simulink model "elec3200lab2"  (R2016a)
settings: Solver=VariableStepAuto  StartTime=0.0  StopTime=2  RelTol=1e-3
libraries: simulink x1
settings Model: Creator=古乔  LastModifiedBy=古乔

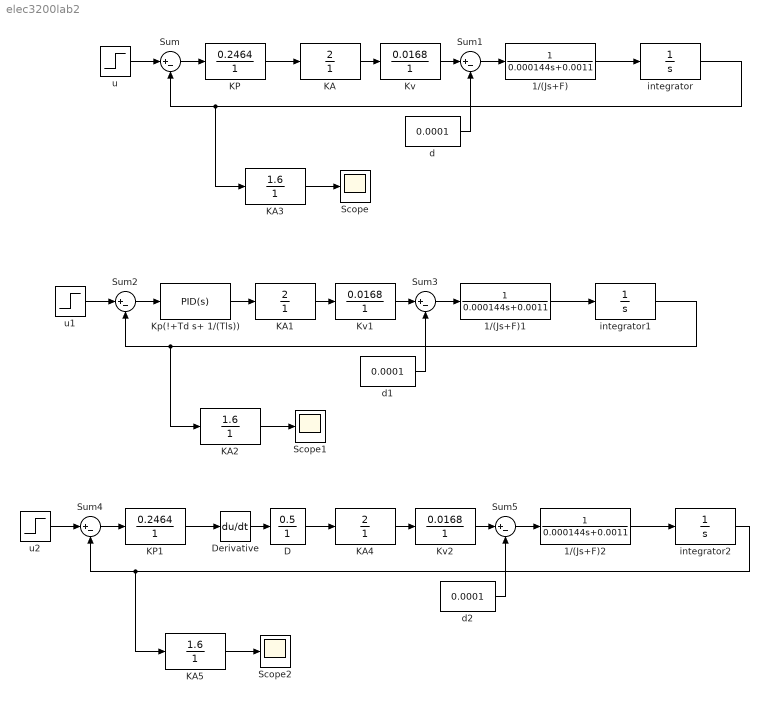
== system elec3200lab2 ==
  " KP" : TransferFcn  Numerator=[0.2464]  Denominator=[1]
  " KP1" : TransferFcn  Numerator=[0.2464]  Denominator=[1]
  1/(Js+F) : TransferFcn  Denominator=[0.000144 0.0011]
  1/(Js+F)1 : TransferFcn  Denominator=[0.000144 0.0011]
  1/(Js+F)2 : TransferFcn  Denominator=[0.000144 0.0011]
  D : TransferFcn  Numerator=[0.5]  Denominator=[1]
  Derivative : Derivative
  KA : TransferFcn  Numerator=[2]  Denominator=[1]
  KA1 : TransferFcn  Numerator=[2]  Denominator=[1]
  KA2 : TransferFcn  Numerator=[1.6]  Denominator=[1]
  KA3 : TransferFcn  Numerator=[1.6]  Denominator=[1]
  KA4 : TransferFcn  Numerator=[2]  Denominator=[1]
  KA5 : TransferFcn  Numerator=[1.6]  Denominator=[1]
  Kp(!+Td s+ 1/(Tls)) : simulink/Continuous/PID Controller  Controller=PID  TimeDomain=Continuous-time  SampleTime=-1  IntegratorMethod=Forward Euler  FilterMethod=Forward Euler  Form=Parallel  UseFilter=on  ControllerParametersSource=internal  P=0.2464  I=0.2464/100  D=0  N=100  InitialConditionSource=internal  InitialConditionForIntegrator=0  InitialConditionForFilter=0  ExternalReset=none  LimitOutput=off  UpperSaturationLimit=inf  LowerSaturationLimit=-inf  LinearizeAsGain=on  AntiWindupMode=none  Kb=1  TrackingMode=off  Kt=1  PParamMin=[]  PParamMax=[]  IParamMin=[]  IParamMax=[]  DParamMin=[]  DParamMax=[]  NParamMin=[]  NParamMax=[]  KbParamMin=[]  KbParamMax=[]  KtParamMin=[]  KtParamMax=[]  POutMin=[]  POutMax=[]  IOutMin=[]  IOutMax=[]  DOutMin=[]  DOutMax=[]  NOutMin=[]  NOutMax=[]  KbOutMin=[]  KbOutMax=[]  KtOutMin=[]  KtOutMax=[]  IntegratorOutMin=[]  IntegratorOutMax=[]  FilterOutMin=[]  FilterOutMax=[]  SumOutMin=[]  SumOutMax=[]  SumI1OutMin=[]  SumI1OutMax=[]  SumI2OutMin=[]  SumI2OutMax=[]  SumI3OutMin=[]  SumI3OutMax=[]  SumDOutMin=[]  SumDOutMax=[]  SaturationOutMin=[]  SaturationOutMax=[]  IntegratorContinuousStateAttributes=''  IntegratorStateMustResolveToSignalObject=off  IntegratorRTWStateStorageClass=Auto  FilterContinuousStateAttributes=''  FilterStateMustResolveToSignalObject=off  FilterRTWStateStorageClass=Auto  DifferentiatorICPrevScaledInput=0  DifferentiatorOutMin=[]  DifferentiatorOutMax=[]
  Kv : TransferFcn  Numerator=[0.0168]  Denominator=[1]
  Kv1 : TransferFcn  Numerator=[0.0168]  Denominator=[1]
  Kv2 : TransferFcn  Numerator=[0.0168]  Denominator=[1]
  Scope : Scope
  Scope1 : Scope
  Scope2 : Scope
  Sum{,1..5} (6 alike) : Sum  Inputs=|+-
  d : Constant  Value=0.0001
  d1 : Constant  Value=0.0001
  d2 : Constant  Value=0.0001
  integrator : TransferFcn  Denominator=[1 0]
  integrator1 : TransferFcn  Denominator=[1 0]
  integrator2 : TransferFcn  Denominator=[1 0]
  u : Step  Time=0  SampleTime=0
  u1 : Step  Time=0  SampleTime=0
  u2 : Step  Time=0  SampleTime=0
  wires:
  u/1 -> Sum/1
  " KP"/1 -> KA/1
  KA/1 -> Kv/1
  1/(Js+F)/1 -> integrator/1
  integrator/1 -> KA3/1, Sum/2
  Sum/1 -> " KP"/1
  Sum1/1 -> 1/(Js+F)/1
  Kv/1 -> Sum1/1
  d/1 -> Sum1/2
  KA3/1 -> Scope/1
  u1/1 -> Sum2/1
  Kp(!+Td s+ 1/(Tls))/1 -> KA1/1
  KA1/1 -> Kv1/1
  1/(Js+F)1/1 -> integrator1/1
  integrator1/1 -> KA2/1, Sum2/2
  Sum2/1 -> Kp(!+Td s+ 1/(Tls))/1
  Sum3/1 -> 1/(Js+F)1/1
  Kv1/1 -> Sum3/1
  d1/1 -> Sum3/2
  KA2/1 -> Scope1/1
  u2/1 -> Sum4/1
  " KP1"/1 -> Derivative/1
  KA4/1 -> Kv2/1
  1/(Js+F)2/1 -> integrator2/1
  integrator2/1 -> KA5/1, Sum4/2
  Sum4/1 -> " KP1"/1
  Sum5/1 -> 1/(Js+F)2/1
  Kv2/1 -> Sum5/1
  d2/1 -> Sum5/2
  KA5/1 -> Scope2/1
  Derivative/1 -> D/1
  D/1 -> KA4/1
